simulink model "halfVehicle2020"  (R2020b)
settings: Solver=ode45  StartTime=0.0  StopTime=10  RelTol=1e-3  EnableMultiTasking=on
values from neighbouring files (symbols this model uses):
  qhalf = halfLinearModel(ms,mus_fl,mus_fr,k_fl,k_fr,c_fl,c_fr,kt_fl,kt_fr,kb,t_f,Ix,actuator)    [Lab_AntiRoll.m]
undefined symbols (not defined in the file or in its folder): hinfK
settings Model: Creator=senameo  LastModifiedBy=DELL
settings DataIOCC: LimitDataPoints=on  SaveFormat=Array  SignalLoggingSaveFormat=ModelDataLogs  ReturnWorkspaceOutputs=off
settings OptimizationCC: InitFltsAndDblsToZero=on  LifeSpan=inf
settings DebuggingCC: AlgebraicLoopMsg=none  SaveWithParameterizedLinksMsg=none  UnderspecifiedInitializationDetection=Classic  MergeDetectMultiDrivingBlocksExec=none  SignalResolutionControl=TryResolveAllWithWarning  MultiTaskDSMMsg=warning  MultiTaskCondExecSysMsg=none  FcnCallInpInsideContextMsg=warning  SFUnexpectedBacktrackingDiag=warning  SFNoUnconditionalDefaultTransitionDiag=warning  SFExecutionAtInitializationDiag=none  ArithmeticOperatorsInVariantConditions=warning
settings HardwareCC: ProdBitPerPointer=32  ProdBitPerSizeT=32  ProdBitPerPtrDiffT=32  ProdLargestAtomicFloat=None  ProdIntDivRoundTo=Undefined  ProdEndianess=Unspecified  ProdWordSize=32  ProdHWDeviceType=32-bit Generic
settings ModelReferenceCC: PropagateSignalLabelsOutOfModel=off
settings SFSimCC: CustomCodeUndefinedFunction=UseInterfaceOnly
settings CodeAppCC: StateflowObjectComments=on
settings GRTTargetCC: TargetFcnLib=ansi_tfl_tmw.mat  TargetLangStandard=C89/C90 (ANSI)  CombineOutputUpdateFcns=off  GRTInterface=on
settings ConfigComp: CovMetricSettings=dw  CovSaveCumulativeToWorkspaceVar=on  CovSaveSingleToWorkspaceVar=on

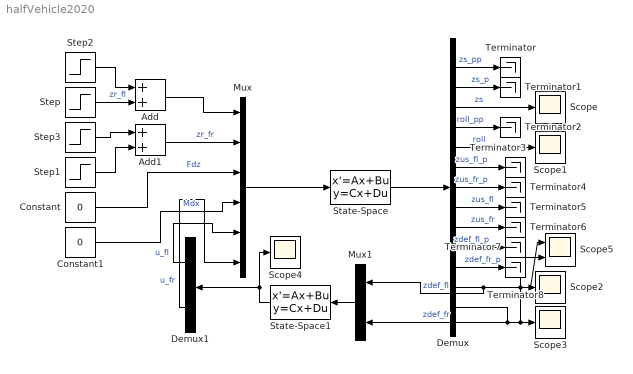
== system halfVehicle2020 ==
  Add : Sum
  Add1 : Sum
  Constant : Constant  Value=0
  Constant1 : Constant  Value=0
  Demux : Demux  Outputs=13
  Demux1 : Demux  Outputs=2
  Mux : Mux  Inputs=6
  Mux1 : Mux  Inputs=2
  Scope{,1..4} (5 alike) : Scope
  Scope5 : Scope  NumInputPorts=2
  State-Space : StateSpace  A=qhalf.a  B=qhalf.b  C=qhalf.c  D=qhalf.d  InitialCondition=0
  State-Space1 : StateSpace  A=hinfK.a  B=hinfK.b  C=hinfK.c  D=hinfK.d  InitialCondition=0
  Step : Step  Time=3  After=-.01  SampleTime=0
  Step1 : Step  Time=8  After=-.01  SampleTime=0
  Step2 : Step  After=.01  SampleTime=0
  Step3 : Step  Time=5  After=.01  SampleTime=0
  Terminator{,1..8} (9 alike) : Terminator
  wires:
  Mux/1 -> State-Space/1
  State-Space/1 -> Demux/1
  Demux/3 -> Scope/1  "zs"
  Demux/1 -> Terminator/1  "zs_pp"
  Demux/2 -> Terminator1/1  "zs_p"
  Demux/4 -> Terminator2/1  "roll_pp"
  Demux/5 -> Scope1/1  "roll"
  Demux/6 -> Terminator3/1  "zus_fl_p"
  Demux/7 -> Terminator4/1  "zus_fr_p"
  Demux/8 -> Terminator5/1  "zus_fl"
  Demux/9 -> Terminator6/1  "zus_fr"
  Demux/10 -> Terminator7/1  "zdef_fl_p"
  Demux/11 -> Terminator8/1  "zdef_fr_p"
  Demux/12 -> Mux1/1, Scope5/1, Scope2/1  "zdef_fl"
  Demux/13 -> Mux1/2, Scope5/2, Scope3/1  "zdef_fr"
  Step/1 -> Add/2  "zr_fl"
  Add1/1 -> Mux/2  "zr_fr"
  Constant/1 -> Mux/3  "Fdz"
  Constant1/1 -> Mux/4  "Mdx"
  Demux1/1 -> Mux/5  "u_fl"
  Demux1/2 -> Mux/6  "u_fr"
  Step2/1 -> Add/1
  Add/1 -> Mux/1
  State-Space1/1 -> Scope4/1, Demux1/1
  Mux1/1 -> State-Space1/1
  Step1/1 -> Add1/2
  Step3/1 -> Add1/1
